simulink model "distortion"  (R2020a)
settings: Solver=FixedStepDiscrete  StartTime=0.0  StopTime=inf  RelTol=1e-3
libraries: dspsnks4 x1, audiosources x1, dspmathops x1
settings Model: Creator=unity  LastModifiedBy=unity
settings SolverCC: AutoInsertRateTranBlk=on
settings DataIOCC: LimitDataPoints=on  SaveOutput=off  SignalLogging=off  SaveTime=off
settings OptimizationCC: LifeSpan=inf
settings DebuggingCC: AlgebraicLoopMsg=error  SingleTaskRateTransMsg=error  AllowSymbolicDim=off  SFUnexpectedBacktrackingDiag=warning  SFNoUnconditionalDefaultTransitionDiag=warning  SFExecutionAtInitializationDiag=none  ArithmeticOperatorsInVariantConditions=warning
settings SFSimCC: SimUseLocalCustomCode=off  CustomCodeUndefinedFunction=UseInterfaceOnly
settings RTWCC: RTWUseLocalCustomCode=off
settings CodeAppCC: StateflowObjectComments=on
settings GRTTargetCC: TargetLangStandard=C89/C90 (ANSI)
settings ConfigComp: CovMetricSettings=dw  CovHtmlReporting=on  CovSaveCumulativeToWorkspaceVar=on  CovSaveSingleToWorkspaceVar=on  CovExternalEMLEnable=off  CovSFcnEnable=off

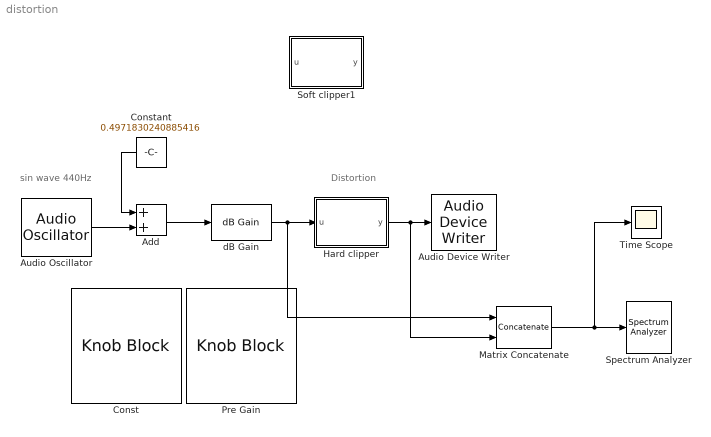
== system distortion ==
  note: sin wave 440Hz
  note: Distortion
  Add : Sum
  Audio Device Writer : dspsnks4/Audio Device Writer  Driver=DirectSound  Device=Default  InheritSampleRate=on  SampleRate=44100  BitDepth=16-bit integer  BufferSize=4096  NumBuffers=10  DefaultOutputChannelMapping=on  OutputChannelMapping=1:2  OutputNumUnderrunSamples=off  DriverIdx=1  DeviceWarnFlag=''
  Audio Oscillator : audiosources/Audio Oscillator  FrequencyPort=off  Frequency=440  AmplitudePort=off  Amplitude=1  DCOffsetPort=off  PhaseOffset=0  DCOffset=0  WidthPort=off  Width=1  DutyCyclePort=off  DutyCycle=0.5  SampsPerFrame=512  Fs=44100  OutputDataType=double  SimulateUsing=Code generation
      settings: SourceProductBaseCode=AU  SignalType=sine
  Const : KnobBlock  ScaleMax=1
  Constant : Constant  Value=0.4971830240885416
  Hard clipper : MATLAB Function  TreatAsAtomicUnit=on
  Matrix Concatenate : Concatenate  Mode=Multidimensional array  ConcatenateDimension=2
  Pre Gain : KnobBlock  ScaleMax=24
  Soft clipper1 : MATLAB Function  TreatAsAtomicUnit=on
  Spectrum Analyzer : SpectrumAnalyzer
  Time Scope : Scope
  dB Gain : dspmathops/dB Gain  dB=6.763328857421875  intype=Amplitude
      settings: SourceProductBaseCode=DS
  wires:
  Matrix Concatenate/1 -> Spectrum Analyzer/1, Time Scope/1
  Constant/1 -> Add/1
  Audio Oscillator/1 -> Add/2
  Add/1 -> dB Gain/1
  dB Gain/1 -> Hard clipper/1(u), Matrix Concatenate/1
  Hard clipper/1(y) -> Matrix Concatenate/2, Audio Device Writer/1

== matlab function distortion/Soft clipper1 ==
  data: u input; y output
function y = fcn(u)
    for i = 1:length(u)
        if (u(i) >= 1)
            u(i) = 2/3;
        elseif (-1 < u(i))
            u(i) = u(i)-u(i)^3/3;
        else
            u(i) = -2/3;
        end
    end
    y = u;

== matlab function distortion/Hard clipper ==
  data: u input; y output
function y = fcn(u)
    for i = 1:length(u)
        if (u(i) >= 1)
            u(i) = 1;
        elseif (-1 < u(i))
            u(i) = u(i);
        else
            u(i) = -1;
        end
    end
    y = u;
